simulink model "CS_PIDVr"  (R2014b)
settings: Solver=ode5  StartTime=0.0  StopTime=Te  FixedStep=Tm  RelTol=1e-3
StopFcn:
  | %salida(simout)
values from neighbouring files (symbols this model uses):
  D = 0    [globales.mat]
  I = 0.6    [globales.mat]
  Kb = 1    [globales.mat]
  P = 0.3    [globales.mat]
  Tm = 0.01    [globales.mat]
  Tp = 5    [globales.mat]    (also in m_CS_PIDVr.m)
  Vf = 50    [globales.mat]    (also in m_CS_PIDVr.m)
  Vi = -50    [globales.mat]    (also in m_CS_PIDVr.m)
undefined symbols (not defined in the file or in its folder): A, B
undefined symbols (not defined in the file): Fcd, Fcv, Nv
settings Model: ExtModeTrigDuration=100000  Creator=Equipo-Servo  LastModifiedBy=E. Rubio
settings DebuggingCC: UnderspecifiedInitializationDetection=Classic  MergeDetectMultiDrivingBlocksExec=none  StateNameClashWarn=warning
settings HardwareCC: ProdIntDivRoundTo=Zero  ProdEndianess=LittleEndian  ProdHWDeviceType=Generic->32-bit x86 compatible
settings RTWCC: SystemTargetFile=rtwin.tlc  TemplateMakefile=rtwin.tmf  Description=Real-Time Windows Target  ProcessScript=rtwin_make_rtw_hook  RTWCompilerOptimization=On
settings CodeAppCC: MaxIdLength=95
settings RTWinTargetCC: TargetLibSuffix=_rtwin.lib  TargetPreCompLibLocation=C:\Program Files\MATLAB\R2014b\toolbox\rtw\targets\rtwin\lib\win64

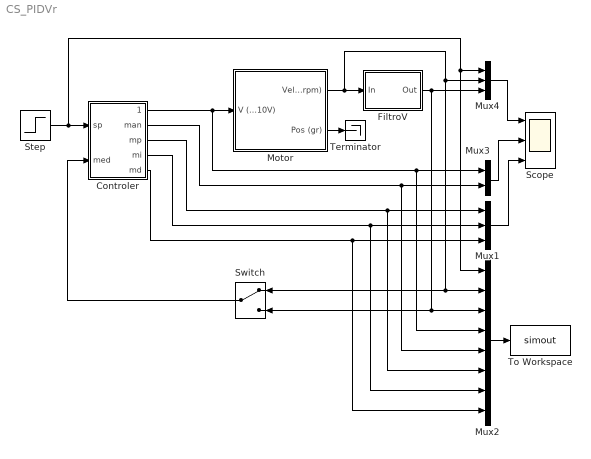
== system CS_PIDVr ==
  Controler : Subsystem  mask{T=Tm, P=P, I=I, Kb=Kb, D=D, Fcd=Fcd}
      mask prompts: T "Período de muestreo"; Kb "Kb (anti windup)"; Fcd "Fcd (Hz)"
      mask init:
      | N = 2*pi*Fcd;
  FiltroV : Subsystem  mask{N=Nv, Fc=Fcv, Fm=1/Tm}
      mask prompts: N "Orden del filtro (Butterworth)"; Fc "Frecuencia de corte (Fc<Fm/2)"; Fm "Frecuencia de muestreo"
      mask init:
      | Fn = Fm/2;   % Frecuencia de Nyquist
      | [B,A] = butter(N,Fc/Fn);
  Motor : Subsystem
  Mux1 : Mux  Inputs=3
  Mux2 : Mux  Inputs=8
  Mux3 : Mux  Inputs=2
  Mux4 : Mux  Inputs=3
  Scope : Scope  NumInputPorts=3
      settings: TimeRange=10  YMin=-20~-10~-10  YMax=30~15~15  SampleTime=Tm
  Step : Step  Time=Tp  Before=Vi  After=Vf  SampleTime=0
  Switch : ManualSwitch
  Terminator : Terminator
  To Workspace : ToWorkspace  VariableName=simout  SaveFormat=Structure With Time  SampleTime=Tm
  wires:
  Mux4/1 -> Scope/1
  Motor/1(Vel (rpm)) -> FiltroV/1(In), Mux2/2, Switch/1, Mux4/2
  Step/1 -> Mux2/1, Mux4/1, Controler/1(sp)
  Mux2/1 -> To Workspace/1
  Controler/1(mans) -> Motor/1(V (+-10V)), Mux2/4, Mux3/1
  FiltroV/1(Out) -> Switch/2, Mux2/3, Mux4/3
  Controler/2(man) -> Mux2/5, Mux3/2
  Controler/3(mp) -> Mux1/1, Mux2/6
  Controler/4(mi) -> Mux1/2, Mux2/7
  Controler/5(md) -> Mux1/3, Mux2/8
  Motor/2(Pos (gr)) -> Terminator/1
  Switch/1 -> Controler/2(med)
  Mux3/1 -> Scope/2
  Mux1/1 -> Scope/3

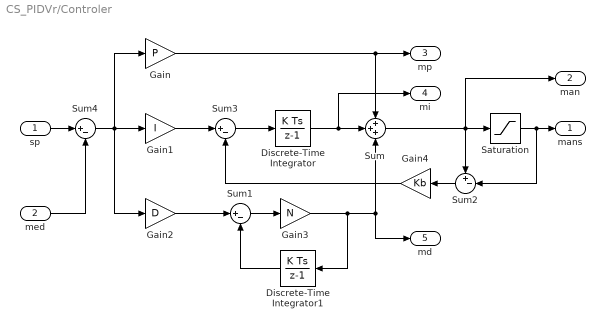
== system CS_PIDVr/Controler ==
  sp : Inport
  med : Inport  Port=2
  Discrete-Time Integrator : DiscreteIntegrator  SampleTime=T
  Discrete-Time Integrator1 : DiscreteIntegrator  SampleTime=T
  Gain : Gain  Gain=P
  Gain1 : Gain  Gain=I
  Gain2 : Gain  Gain=D
  Gain3 : Gain  Gain=N
  Gain4 : Gain  Gain=Kb
  Saturation : Saturate  UpperLimit=10  LowerLimit=-10
  Sum : Sum  Inputs=+++
  Sum1 : Sum  Inputs=|+-
  Sum2 : Sum  Inputs=+-|
  Sum3 : Sum  Inputs=|+-
  Sum4 : Sum  Inputs=|+-
  mans : Outport
  man : Outport  Port=2
  mp : Outport  Port=3
  mi : Outport  Port=4
  md : Outport  Port=5
  wires:
  Sum/1 -> man/1, Sum2/1, Saturation/1
  Saturation/1 -> Sum2/2, mans/1
  Gain/1 -> Sum/1, mp/1
  Discrete-Time Integrator/1 -> mi/1, Sum/2
  sp/1 -> Sum4/1
  Sum1/1 -> Gain3/1
  Gain2/1 -> Sum1/1
  Discrete-Time Integrator1/1 -> Sum1/2
  Gain3/1 -> md/1, Sum/3, Discrete-Time Integrator1/1
  Sum2/1 -> Gain4/1
  Sum3/1 -> Discrete-Time Integrator/1
  Gain1/1 -> Sum3/1
  Gain4/1 -> Sum3/2
  Sum4/1 -> Gain2/1, Gain/1, Gain1/1
  med/1 -> Sum4/2

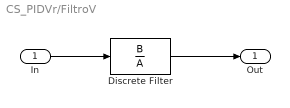
== system CS_PIDVr/FiltroV ==
  In : Inport
  Discrete Filter : DiscreteFilter  Numerator=B  Denominator=A  SampleTime=1/Fm
  Out : Outport
  wires:
  Discrete Filter/1 -> Out/1
  In/1 -> Discrete Filter/1

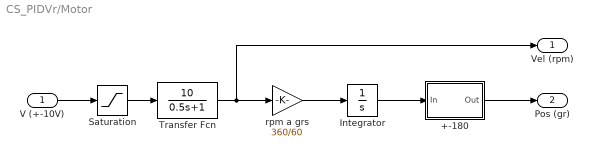
== system CS_PIDVr/Motor ==
  V (+-10V) : Inport
  +-180 : Subsystem
  Integrator : Integrator  InitialCondition=180  UpperSaturationLimit=180  LowerSaturationLimit=-180
  Saturation : Saturate  UpperLimit=10  LowerLimit=-10
  Transfer Fcn : TransferFcn  Numerator=[10]  Denominator=[0.5 1]
  rpm a grs : Gain  Gain=360/60
  Vel (rpm) : Outport
  Pos (gr) : Outport  Port=2
  wires:
  V (+-10V)/1 -> Saturation/1
  Transfer Fcn/1 -> Vel (rpm)/1, rpm a grs/1
  Integrator/1 -> +-180/1(In)
  Saturation/1 -> Transfer Fcn/1
  +-180/1(Out) -> Pos (gr)/1
  rpm a grs/1 -> Integrator/1

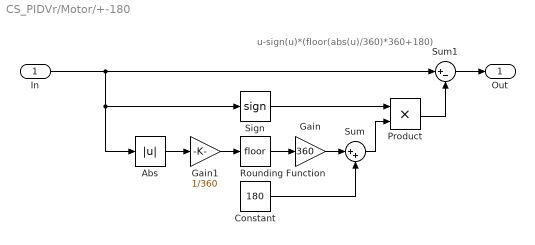
== system CS_PIDVr/Motor/+-180 ==
  note: u-sign(u)*(floor(abs(u)/360)*360+180)
  In : Inport
  Abs : Abs
  Constant : Constant  Value=180
  Gain : Gain  Gain=360
  Gain1 : Gain  Gain=1/360
  Product : Product
  Rounding Function : Rounding
  Sign : Signum
  Sum : Sum  Inputs=|++
  Sum1 : Sum  Inputs=|+-
  Out : Outport
  wires:
  Sum/1 -> Product/2
  Constant/1 -> Sum/2
  Sign/1 -> Product/1
  Gain1/1 -> Rounding Function/1
  Gain/1 -> Sum/1
  Rounding Function/1 -> Gain/1
  Sum1/1 -> Out/1
  Abs/1 -> Gain1/1
  Product/1 -> Sum1/2
  In/1 -> Abs/1, Sign/1, Sum1/1
